simulink model "KitGewerk2_v1_2_robi"  (R2014a)
settings: Solver=ode3  StartTime=0.0  StopTime=inf  FixedStep=0.005  RelTol=1e-3
undefined symbols (not defined in the file): Com1, none
libraries: slrtlib x14, dspswit3 x1, xpcseriallib x1
(part 2 of 2)

== matlab function KitGewerk2_v1_2_robi/Robotino/assemble robotino response ==
  data: v_x_in input; robotino_response output; v_y_in input; v_theta_in input; distance_measuring_sensors_in input; bumper_in input; light_barrier_in input; slider_in input
%%%%%%%%%%%%%%%%%%%%%%%%%%%%%%%%%%%%%%%%%%%%%%%%%%%%%%%%%%%%%%%%%%%%%%%%%%%
% Assembly of robot data in a vector of 34 elements.                      %
%                                                                         %
% inputs:   longitudinal, lateral and rotational velocity (in mm/s),      %
%           shaft positions of the three motors (4 elements per motor),   %
%           running times of the three motors (3 elements per motor),     %
%           values of the nine IR-sensors (in mm),                        %
%           bumper collision (1 = no collision;                           %
%                             0 = collision)                              %
% outputs:  vector containing assembled input data                        %
%%%%%%%%%%%%%%%%%%%%%%%%%%%%%%%%%%%%%%%%%%%%%%%%%%%%%%%%%%%%%%%%%%%%%%%%%%%
function robotino_response = fcn(v_x_in, v_y_in, v_theta_in, ...
                                 distance_measuring_sensors_in, ...
                                 bumper_in, light_barrier_in, slider_in)
                                 % motor_positions_in, time_bytes_in, ...)
robotino_response = [light_barrier_in, slider_in, v_x_in, v_y_in, ...
                     v_theta_in, ...%motor_positions_in, time_bytes_in, ...
                     distance_measuring_sensors_in, bumper_in]';

== matlab function KitGewerk2_v1_2_robi/Robotino/light barrier & slider ==
  data: di03_bump_in input; light_barrier output; slider output
function [light_barrier, slider] = fcn(di03_bump_in)
%%%%%%%%%%%%%%%%%%%%%%%%%%%%%%%%%%%%%%%%%%%%%%%%%%%%%%%%%%%%%%%%%%%%%%%%%%%
% di03_bump_in = 0 alternatively 12 ->  no light barrier activation       %
%                                       no slider activation              %
% di03_bump_in = 13                 ->  only light barrier activation     %
% di03_bump_in = 14                 ->  only slider activation            %
% di03_bump_in = 15                 ->  light barrier activation          %
%                                       slider activation                 %
%%%%%%%%%%%%%%%%%%%%%%%%%%%%%%%%%%%%%%%%%%%%%%%%%%%%%%%%%%%%%%%%%%%%%%%%%%%
% function [light_barrier, slider] = fcn(di03_bump_in)
% bin = dec2bin(di03_bump_in);
% if bin(3) == 1
%     light_barrier = 1;
% else
%     light_barrier = 0;
% end
% if bin(4) == 1
%     slider = 1;
% else
%     slider = 0;
% end
if     di03_bump_in == 13
    light_barrier = 1;
    slider        = 0;
elseif di03_bump_in == 14
    light_barrier = 0;
    slider        = 1;
elseif di03_bump_in == 15
    light_barrier = 1;
    slider        = 1;
else
    light_barrier = 0;
    slider        = 0;
end

== matlab function KitGewerk2_v1_2_robi/Begrenzung1 ==
  data: win input; wout output
function wout = fnc(win)
wert= zeros(1);
if win > 500
    wert = 500;
else
    wert = win;
end
wout = wert;

== matlab function KitGewerk2_v1_2_robi/Begrenzung2 ==
  data: win input; wout output
function wout = fnc(win)
wert= zeros(1);
if win > 3,14
    wert = 3,14;
else
    wert = win;
end
wout = wert;

== matlab function KitGewerk2_v1_2_robi/Gewerk_2/Kollisionserkennung ==
  data: d_Abstand input; b_stop output boolean; ad_Abstandssensor input
function b_stop = fcn(d_Abstand,ad_Abstandssensor)
b_stop=false;
if sum(isnan(ad_Abstandssensor))==9 % nan = kein Hinderniss
    % kein Hinderniss   
    b_stop= false; 
else
    % Hinderniss entdeckt, min. ein Sensor(kein nan)
    if ( (ad_Abstandssensor(1)<d_Abstand) || (ad_Abstandssensor(2)<d_Abstand) || (ad_Abstandssensor(3)<d_Abstand) || ...
         (ad_Abstandssensor(4)<d_Abstand) ||(ad_Abstandssensor(5)<d_Abstand) ||(ad_Abstandssensor(6)<d_Abstand) || ...
         (ad_Abstandssensor(7)<d_Abstand) || (ad_Abstandssensor(8)<d_Abstand) ||(ad_Abstandssensor(9)<d_Abstand)) 

    b_stop= true;
    end
end

== matlab function KitGewerk2_v1_2_robi/Gewerk_2/MATLAB Function ==
  data: ad_PL input; d_Y_soll output double; d_X_soll output double; d_Phi_soll output double; d_V_Max_soll output double; int_I input
function [d_Y_soll,d_X_soll,d_Phi_soll,d_V_Max_soll]= fcn(ad_PL,int_I)

int_I=int_I+1; %Offset, da Zeilenindex bei 1 beginnt

d_Y_soll= ad_PL(int_I,1);
d_X_soll= ad_PL(int_I,2);
d_Phi_soll= ad_PL(int_I,3);
d_V_Max_soll= ad_PL(int_I,4);
